simulink model "robot_3gdl_PD"  (R2025b)
settings: Solver=VariableStepAuto  StartTime=0.0  StopTime=10  RelTol=1e-3
settings Model: Creator=al177  LastModifiedBy=al177

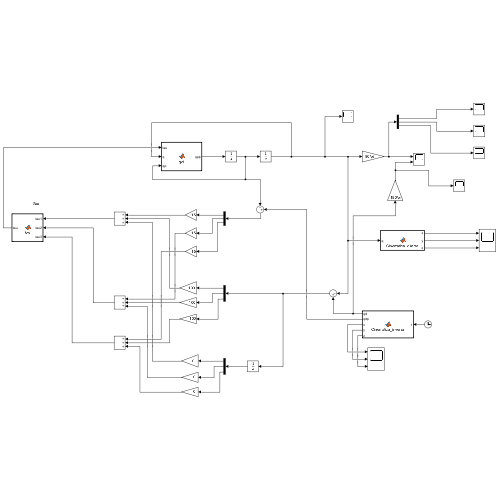
[thumbnail: Simulink's stored preview of the top-level diagram]
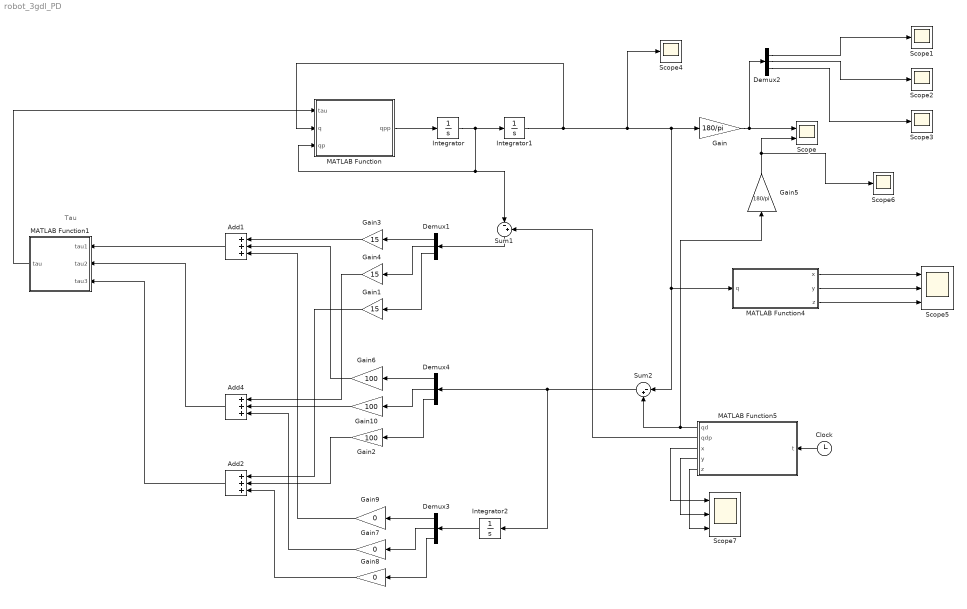
== system robot_3gdl_PD ==
  note: Tau
  Add1 : Sum  Inputs=+++
  Add2 : Sum  Inputs=+++
  Add4 : Sum  Inputs=+++
  Clock : Clock
  Demux{1..4} (4 alike) : Demux  Outputs=3
  Gain : Gain  Gain=180/pi
  Gain1 : Gain  Gain=15
  Gain10 : Gain  Gain=100
  Gain2 : Gain  Gain=100
  Gain3 : Gain  Gain=15
  Gain4 : Gain  Gain=15
  Gain5 : Gain  Gain=180/pi
  Gain6 : Gain  Gain=100
  Gain7 : Gain  Gain=0
  Gain8 : Gain  Gain=0
  Gain9 : Gain  Gain=0
  Integrator : Integrator  InitialCondition=[0;0;0]
  Integrator1 : Integrator  InitialCondition=[pi/6;pi/4;-pi/3]
  Integrator2 : Integrator  InitialCondition=[0;0;0]
  MATLAB Function : MATLAB Function  TreatAsAtomicUnit=on
  MATLAB Function1 : MATLAB Function  TreatAsAtomicUnit=on
  MATLAB Function4 : MATLAB Function  TreatAsAtomicUnit=on
  MATLAB Function5 : MATLAB Function  TreatAsAtomicUnit=on
  Scope : Scope  NumInputPorts=2
      settings: ActiveDisplayYMinimum=-135.17452320744422  ActiveDisplayYMaximum=115.0193914674938
  Scope{1..4,6} (5 alike) : Scope
      Scope1 settings: ActiveDisplayYMinimum=-1  ActiveDisplayYMaximum=1
      Scope2 settings: ActiveDisplayYMinimum=-14.816570606469632  ActiveDisplayYMaximum=16.928522882066108  DataLoggingVariableName=ScopeData2
      Scope3 settings: ActiveDisplayYMinimum=-14.816570606469632  ActiveDisplayYMaximum=16.928522882066108  DataLoggingVariableName=ScopeData3
      Scope4 settings: ActiveDisplayYMinimum=-0.41771144886533496  ActiveDisplayYMaximum=0.30859430648296182  DataLoggingVariableName=q  DataLoggingSaveFormat=Array
      Scope6 settings: ActiveDisplayYMinimum=-1  ActiveDisplayYMaximum=1  DataLoggingVariableName=ScopeData4
  Scope5 : Scope  NumInputPorts=3
      settings: ActiveDisplayYMinimum=-1  ActiveDisplayYMaximum=1  DataLoggingVariableName=pos
  Scope7 : Scope  NumInputPorts=3
      settings: ActiveDisplayYMinimum=-1  ActiveDisplayYMaximum=1  DataLoggingVariableName=posd
  Sum1 : Sum  Inputs=|-+
  Sum2 : Sum  Inputs=|-+
  wires:
  Demux1/2 -> Gain4/1
  Add4/1 -> MATLAB Function1/2(tau2)
  Demux4/2 -> Gain10/1
  Gain10/1 -> Add4/2
  Demux2/2 -> Scope2/1
  MATLAB Function1/1(tau) -> MATLAB Function/1(tau)
  Gain6/1 -> Add1/2
  Demux1/1 -> Gain3/1
  Gain4/1 -> Add4/1
  Integrator/1 -> Sum1/1, MATLAB Function/3(qp), Integrator1/1
  Demux4/3 -> Gain2/1
  Gain/1 -> Scope/1, Demux2/1
  Demux1/3 -> Gain1/1
  Sum2/1 -> Demux4/1, Integrator2/1
  Demux2/1 -> Scope1/1
  MATLAB Function/1(qpp) -> Integrator/1
  Sum1/1 -> Demux1/1
  Add2/1 -> MATLAB Function1/3(tau3)
  Gain2/1 -> Add2/2
  Add1/1 -> MATLAB Function1/1(tau1)
  Demux4/1 -> Gain6/1
  Integrator1/1 -> Scope4/1, Gain/1, MATLAB Function4/1(q), Sum2/1, MATLAB Function/2(q)
  Gain1/1 -> Add2/1
  Gain5/1 -> Scope6/1, Scope/2
  Demux2/3 -> Scope3/1
  Gain3/1 -> Add1/1
  MATLAB Function5/1(qd) -> Gain5/1, Sum2/2
  MATLAB Function5/2(qdp) -> Sum1/2
  Clock/1 -> MATLAB Function5/1(t)
  MATLAB Function5/3(x) -> Scope7/1
  MATLAB Function5/4(y) -> Scope7/2
  MATLAB Function5/5(z) -> Scope7/3
  Integrator2/1 -> Demux3/1
  MATLAB Function4/3(z) -> Scope5/3
  MATLAB Function4/2(y) -> Scope5/2
  MATLAB Function4/1(x) -> Scope5/1
  Demux3/3 -> Gain8/1
  Demux3/1 -> Gain9/1
  Demux3/2 -> Gain7/1
  Gain9/1 -> Add1/3
  Gain7/1 -> Add4/3
  Gain8/1 -> Add2/3

== matlab function robot_3gdl_PD/MATLAB Function1 ==
  data: tau1 input; tau output; tau2 input; tau3 input
function tau = fcn(tau1, tau2, tau3)

tau = [tau1;tau2;tau3];

== matlab function robot_3gdl_PD/MATLAB Function ==
  data: tau input; qpp output; q input; qp input
function qpp = gdl(tau, q, qp)

q1 = q(1);   q2 = q(2);   q3 = q(3);
q1p = qp(1); q2p = qp(2); q3p = qp(3);

T1 = tau(1); T2 = tau(2); T3 = tau(3);

l1 = 0.4; lc1 = 0.2;
l2 = 1.0; lc2 = 0.5;
l3 = 1.0; lc3 = 0.5;
m1 = 1; m2 = 1; m3 = 1;
I1 = 0.001; I2 = 0.001; I3 = 0.001;
g = 9.81;

fx = 0; fy = 0; fz = -50;

% Ejes de rotación 
s1 = [0; 0; 1; 0; 0; 0]; 
s2 = [0; 0; 1; 0; 0; 0]; 
s3 = [0; 0; 1; 0; 0; 0]; 

% Transformaciones locales espaciales 
X1 = rotz(q1);
X2 = rotz(q2) * rotx(pi/2) * xlt([0; 0; l1]); 
X3 = rotz(q3) * xlt([l2; 0; 0]);
X4 = xlt([l3; 0; 0]); 

% Matrices de Inercia Espacial
I1_e = mcI(m1, [0; 0; lc1], diag([I1, I1, I1]));
I2_e = mcI(m2, [lc2; 0; 0], diag([I2, I2, I2]));
I3_e = mcI(m3, [lc3; 0; 0], diag([I3, I3, I3]));

% Condición inicial                                          
v0 = zeros(6,1);
a0 = [0; 0; 0; 0; 0; g]; 

% Matrices de rotación
R1 = X1(1:3, 1:3);
R2 = X2(1:3, 1:3);
R3 = X3(1:3, 1:3);

% Matriz de rotación del marco 4 al marco 0
R_0_4 = R3 * R2 * R1; 
f_loc3 = R_0_4 * [fx; fy; fz];
f4 = [0; 0; 0; f_loc3];

% Pasada 1: Cinemática hacia adelante 
v1 = X1*v0 + s1*q1p;
c1 = crm(v1)*(s1*q1p);
p1 = crf(v1)*(I1_e*v1);

v2 = X2*v1 + s2*q2p;
c2 = crm(v2)*(s2*q2p);
p2 = crf(v2)*(I2_e*v2);

v3 = X3*v2 + s3*q3p;
c3 = crm(v3)*(s3*q3p);
p3 = crf(v3)*(I3_e*v3);

% Pasada 2: Inercia articulada hacia atrás 
I3_A = I3_e;
p3_A = p3 - X4'*f4; 
U3 = I3_A*s3;
D3 = s3'*U3;
u_3 = T3 - s3'*p3_A;
I3a = I3_A - (U3*U3')/D3;
p3a = p3_A + I3a*c3 + U3*(u_3/D3);

I2_A = I2_e + X3'*I3a*X3;
p2_A = p2 + X3'*p3a;
U2 = I2_A*s2;
D2 = s2'*U2;
u_2 = T2 - s2'*p2_A;
I2a = I2_A - (U2*U2')/D2;
p2a = p2_A + I2a*c2 + U2*(u_2/D2);

I1_A = I1_e + X2'*I2a*X2;
p1_A = p1 + X2'*p2a; 
U1 = I1_A*s1;
D1 = s1'*U1;
u_1 = T1 - s1'*p1_A;

% Pasada 3: Aceleraciones articuladas hacia adelante 
a1_p = X1*a0 + c1;
q1pp = (u_1 - U1'*a1_p)/D1;
a1   = a1_p + s1*q1pp;

a2_p = X2*a1 + c2;
q2pp = (u_2 - U2'*a2_p)/D2;
a2   = a2_p + s2*q2pp;

a3_p = X3*a2 + c3;
q3pp = (u_3 - U3'*a3_p)/D3;

qpp = [q1pp; q2pp; q3pp];

end

== matlab function robot_3gdl_PD/MATLAB Function4 ==
  data: q input; x output; y output; z output
function [x, y, z] = Cinematica_directa(q)

q1 = q(1);
q2 = q(2);
q3 = q(3); 

l1 = 0.4; 
l2 = 1.0; 
l3 = 1.0; 

x = cos(q1)*(l3*cos(q2 + q3) + l2*cos(q2));
y = sin(q1)*(l3*cos(q2 + q3) + l2*cos(q2));
z = l1 + l3*sin(q2 + q3) + l2*sin(q2);


end

== matlab function robot_3gdl_PD/MATLAB Function5 ==
  data: t input; qd output; qdp output; x output; y output; z output
function [qd, qdp, x, y, z] = Cinematica_inversa(t)
    l1 = 0.4; l2 = 1.0; l3 = 1.0;

    % Parámetros de la trayectoria circular (Plano X-Y)
    xc = 1.2; yc = 0.8; zc = 0.5; R = 0.25; 
    f = 0.2; 
    omega = (2*pi) * f;

    % Posición deseada (Mismo plano Y-Z que en Python)
    x_d = [xc + R*cos(omega*t); 
           yc + R*sin(omega*t); 
           zc];
    
    % Velocidad deseada (Derivada exacta de x_d)
    xdp_d = [ -R*omega*sin(omega*t); 
              R*omega*cos(omega*t);
              0.0];

    x = x_d(1); y = x_d(2); z = x_d(3);

    % Cinemática inversa de posición 
    q1 = atan2(y, x);
    r = sqrt(x^2 + y^2);
    zp = z - l1;

    D = (r^2 + zp^2 - l2^2 - l3^2) / (2 * l2 * l3);
    %D = max(-1.0, min(1.0, D)); 

    s3 = -sqrt(1 - D^2); % codo arriba
    q3 = atan2(s3, D);
    q2 = atan2(zp, r) - atan2(l3 * s3, l2 + l3 * D);

    qd = [q1; q2; q3];

    % Jacobiano analítico
    rp_q2p = -l2*sin(q2) - l3*sin(q2 + q3);
    rp_q3p = -l3*sin(q2 + q3);

    J = [ -r*sin(q1), rp_q2p*cos(q1), rp_q3p*cos(q1);
           r*cos(q1), rp_q2p*sin(q1), rp_q3p*sin(q1);
           0,         l2*cos(q2) + l3*cos(q2 + q3), l3*cos(q2 + q3) ];

    % Cinemática inversa de velocidad
    qdp = J \ xdp_d;
end
